simulink model "rtwdemo_filepart"  (Simulink 6.0)
settings: Solver=FixedStepDiscrete  StartTime=0.0  StopTime=10.0  RelTol=1e-3
libraries: rtwdemowidgets x2
settings Model: Creator=The MathWorks Inc.  LastModifiedBy=batserve  ExtModeAutoUpdateStatusClock=off
settings DataIOCC: SaveOutput=off  SaveTime=off  SignalLoggingName=sigsOut
settings OptimizationCC: InlineParams=on  EnforceIntegerDowncast=off  StateBitsets=on  DataBitsets=on  UseTempVars=on
settings DebuggingCC: CheckExecutionContextPreStartOutputMsg=on  CheckExecutionContextRuntimeOutputMsg=on  SolverPrmCheckMsg=none
settings RTWCC: TLCOptions=-p0 -aWarnNonSaturatedBlocks=0  GenerateReport=on  RTWVerbose=off  ProcessScript=grt_make_rtw_hook  LaunchReport=on
settings CodeAppCC: ForceParamTrailComments=on  PrefixModelToSubsysFcnNames=off
settings GRTTargetCC: MatFileLogging=off

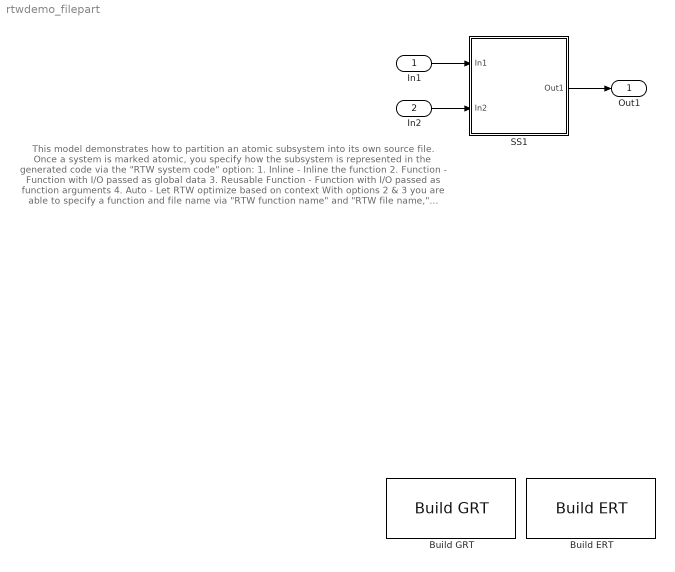
== system rtwdemo_filepart ==
  note: This model demonstrates how to partition an atomic subsystem into its own source file.  Once a system
      | is marked atomic, you specify how the subsystem is represented in the generated code via the "RTW
      | system code" option:
      |
      | 1. Inline            - Inline the function
      | 2. Function          - Function with I/O passed as global data
      | 3. Reusable Function - Function with I/O passed as function arguments
      | 4. Auto              - Let RTW optimize based on context
      |
      | With options 2 & 3 you are able to specify a function and file name via "RTW function name" and "RTW
      | file name," respectively.  Here, SS1 is configured as "Function" with function name "myfun" and file
      | name "myfile."
      |
      | To view the subsystem parameters, right-click on the subsystem block and choose "SubSystem
      | Parameters..."
      |
      | NOTE: This capability only partitions the code for a subsystem.  The data is declared and "owned" by
      | the parent model.  For full system encapsulation (i.e., data and function) use Model Reference.
  In1 : Inport  Port=1  LatchInput=off
  In2 : Inport  Port=2  LatchInput=off
  Build ERT : rtwdemowidgets/Build ERT  attrib_overrides={}
  Build GRT : rtwdemowidgets/Build GRT  attrib_overrides={}
  SS1 : Subsystem  TreatAsAtomicUnit=on  PropExecContextAcrossSSBoundary=on  RTWFcnName=myfun  RTWFileName=myfile
      settings: RTWSystemCode=Function  RTWFcnNameOpts=User specified  RTWFileNameOpts=User specified
  Out1 : Outport
  wires:
  SS1/1(Out1) -> Out1/1
  In2/1 -> SS1/2(In2)
  In1/1 -> SS1/1(In1)

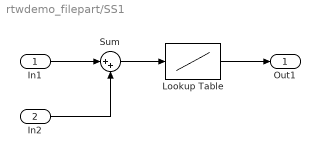
== system rtwdemo_filepart/SS1 ==
  In1 : Inport  Port=1  LatchInput=off
  In2 : Inport  Port=2  LatchInput=off
  Lookup Table : Lookup  DialogController=Simulink.DDGSource  InputValues=[-5:5]  OutputValues=tanh([-5:5])
  Sum : Sum  Inputs=|++
  Out1 : Outport
  wires:
  In1/1 -> Sum/1
  Lookup Table/1 -> Out1/1
  In2/1 -> Sum/2
  Sum/1 -> Lookup Table/1
